simulink library "PowerFlowLib"  (Simulink 8.1)
settings: Solver=ode45  StartTime=0.0  StopTime=10.0  RelTol=1e-3
undefined symbols (not defined in the file or in its folder): Air, AirProp, C, F1, F2, Fanmap, Fld1, Fld2, Fluid, fueltankdata, HydProp, HydraulicLoad, IBFD_exc, L, LoadFluidProps, magnitude, MSSN, n_alghts, PumpProp, pwr_alghts, R_fd_exc, Rcore, Ts, VBFD_exc
libraries: PowerFlowLib x35, simulink x19, powerlib_extras x2, dspstat3 x2
(part 10 of 12)

== system PowerFlowLib/Energy & Power Systems/Electrical/Machines/Synchronous Machine P.U. dq0/Generator Power Loss ==
  Ed : Inport
  Eq : Inport  Port=2
  Id : Inport  Port=3
  Iq : Inport  Port=4
  Te : Inport  Port=5
  w/ws : Inport  Port=6
  Bus Creator : BusCreator  Inputs=6
  Gain1 : Gain  Gain=SB
  Gain2 : Gain  Gain=SB
  Gain3 : Gain  Gain=SB
  Product : Product  RndMeth=Zero
  Product1 : Product  RndMeth=Zero
  Product2 : Product  RndMeth=Zero
  Sum1 : Sum  Inputs=-+
  Sum2 : Sum
  PE : Outport
  PM : Outport  Port=2
  PLOSS : Outport  Port=3
  m : Outport  Port=4
  wires:
  Gain3/1 -> PM/1
  Gain1/1 -> PE/1
  Gain2/1 -> PLOSS/1
  Bus Creator/1 -> m/1
  [nu] -> Bus Creator/6  "nu"
  [Te] -> Bus Creator/5  "Te"
  [Iq] -> Bus Creator/4  "Iq"
  [Eq] -> Bus Creator/3  "Vq"
  [Id] -> Bus Creator/2  "Id"
  [Ed] -> Bus Creator/1  "Vd"
  Sum1/1 -> Gain2/1
  Product2/1 -> Gain3/1, Sum1/2
  Sum2/1 -> Gain1/1, Sum1/1
  Product1/1 -> Sum2/2
  Product/1 -> Sum2/1
  [nu] -> Product2/2
  [Te] -> Product2/1
  [Iq] -> Product1/2
  [Eq] -> Product1/1
  [Id] -> Product/2
  [Ed] -> Product/1
  w/ws/1 -> [nu]
  Te/1 -> [Te]
  Iq/1 -> [Iq]
  Id/1 -> [Id]
  Eq/1 -> [Eq]
  Ed/1 -> [Ed]

== system PowerFlowLib/Energy & Power Systems/Electrical/Machines/Synchronous Machine P.U. dq0/Generator Power Loss1 ==
  Ploss : Inport
  Tamb : Inport  Port=2
  Gain1 : Gain  Gain=1/mc_gen
  Heat Trasnfer : Subsystem
  Integrator : Integrator  InitialConditionSource=external
  Sum : Sum  Inputs=|+-
  Ts : Outport
  Pdiss : Outport  Port=2
  wires:
  Gain1/1 -> Integrator/1
  Heat Trasnfer/1(Pdiss) -> Pdiss/1, Sum/2
  Ploss/1 -> Sum/1
  Sum/1 -> Gain1/1
  Integrator/1 -> Heat Trasnfer/2(Ts), Ts/1
  Tamb/1 -> Heat Trasnfer/1(Tamb), Integrator/2

== system PowerFlowLib/Energy & Power Systems/Electrical/Machines/Synchronous Machine P.U. dq0/Stator Voltage ==
  Id : Inport
  Iq : Inport  Port=2
  Eq1 : Inport  Port=3
  Ed1 : Inport  Port=4
  Phi_1d : Inport  Port=5
  Phi_2q : Inport  Port=6
  w/ws : Inport  Port=7
  Gain : Gain  Gain=(Xq2 - Xls)/(Xq1 - Xls)
  Gain1 : Gain  Gain=(Xq1 - Xq2)/(Xq1 - Xls)
  Gain2 : Gain  Gain=(Xq2 - Xd2)
  Gain3 : Gain  Gain=(Xd2 - Xls)/(Xd1 - Xls)
  Gain4 : Gain  Gain=(Xd1 - Xd2)/(Xd1 - Xls)
  Gain5 : Gain  Gain=Rs
  Gain6 : Gain  Gain=Xd2+XTL
  Gain7 : Gain  Gain=Rs+RTL
  Gain8 : Gain  Gain=Xd2+XTL
  Product{,1..3} (4 alike) : Product  RndMeth=Zero
  Sum : Sum
  Sum1 : Sum  Inputs=+-+
  Sum2 : Sum  Inputs=--+
  Sum3 : Sum  Inputs=-++
  Ed : Outport
  Eq : Outport  Port=2
  wires:
  Gain7/1 -> Sum2/2
  Product3/1 -> Sum2/1
  Sum2/1 -> Eq/1  "Vq"
  Sum3/1 -> Ed/1  "Vd"
  Product2/1 -> Sum3/3
  Gain2/1 -> Sum1/3
  Product1/1 -> Sum3/2
  Gain8/1 -> Product3/1
  Gain5/1 -> Sum3/1
  Gain6/1 -> Product2/2
  Id/1 -> Gain8/1, Gain5/1
  Product/1 -> Sum2/3
  w/ws/1 -> Product2/1, Product3/2, Product/2, Product1/2
  Sum1/1 -> Product1/1
  Sum/1 -> Product/1
  Gain1/1 -> Sum1/2
  Gain/1 -> Sum1/1
  Gain3/1 -> Sum/1
  Gain4/1 -> Sum/2
  Phi_1d/1 -> Gain4/1
  Eq1/1 -> Gain3/1
  Iq/1 -> Gain2/1, Gain7/1, Gain6/1
  Phi_2q/1 -> Gain1/1
  Ed1/1 -> Gain/1

== system PowerFlowLib/Energy & Power Systems/Electrical/Systems/Gen Bus w/ APU switch/VOLTAGE FAULT DETECTION LOGIC ==
  note: This input determines the start of voltage monitoring
  In1 : Inport
  Constant1 : Constant  Value=LOWVLIMIT
  Constant2 : Constant  Value=UPVLIMIT
  Logical Operator : Logic  Operator=OR  AllPortsSameDT=off  OutDataTypeStr=boolean
  Logical Operator1 : Logic  Operator=NAND  AllPortsSameDT=off  OutDataTypeStr=boolean
  Relational Operator : RelationalOperator  Operator=<=  OutDataTypeStr=boolean  ZeroCross=off
  Relational Operator1 : RelationalOperator  OutDataTypeStr=boolean  ZeroCross=off
  Fault Signal  (Acitve Low) : Outport
  wires:
  Logical Operator1/1 -> Fault Signal  (Acitve Low)/1
  In1/1 -> Relational Operator1/1, Relational Operator/1
  [enable] -> Logical Operator1/2
  Logical Operator/1 -> Logical Operator1/1
  Relational Operator1/1 -> Logical Operator/2
  Relational Operator/1 -> Logical Operator/1
  Constant2/1 -> Relational Operator1/2
  Constant1/1 -> Relational Operator/2

== system PowerFlowLib/Energy & Power Systems/Electrical/Systems/Generation Unit Sync-Sync/Chopper (Averaged) ==
  vin : Inport
  q : Inport  Port=2
  Temperature : Inport  Port=3
  1/R : Gain  Gain=1/(R_fd_exc*VBFD_exc/IBFD_exc)/100/2*3/100  SaturateOnIntegerOverflow=on  OutDataTypeStr=Inherit: Same as input  ParamDataTypeStr=Inherit: Same as input
  Divide : Product  Inputs=*/
  Dot Product : DotProduct  InputSameDT=on  OutDataTypeStr=Inherit: Inherit via internal rule
  Dot Product1 : DotProduct  InputSameDT=on  OutDataTypeStr=Inherit: Inherit via internal rule
  Gain2 : Gain  Gain=1000*2/3
  Saturation : Saturate  UpperLimit=1  LowerLimit=0
  iout : Outport
  iin : Outport  Port=2
  wires:
  Dot Product1/1 -> iin/1
  Saturation/1 -> Dot Product1/2, Dot Product/2
  Dot Product/1 -> 1/R/1
  q/1 -> Saturation/1
  vin/1 -> Dot Product/1
  Gain2/1 -> Dot Product1/1, iout/1
  1/R/1 -> Divide/1
  Temperature/1 -> Divide/2
  Divide/1 -> Gain2/1

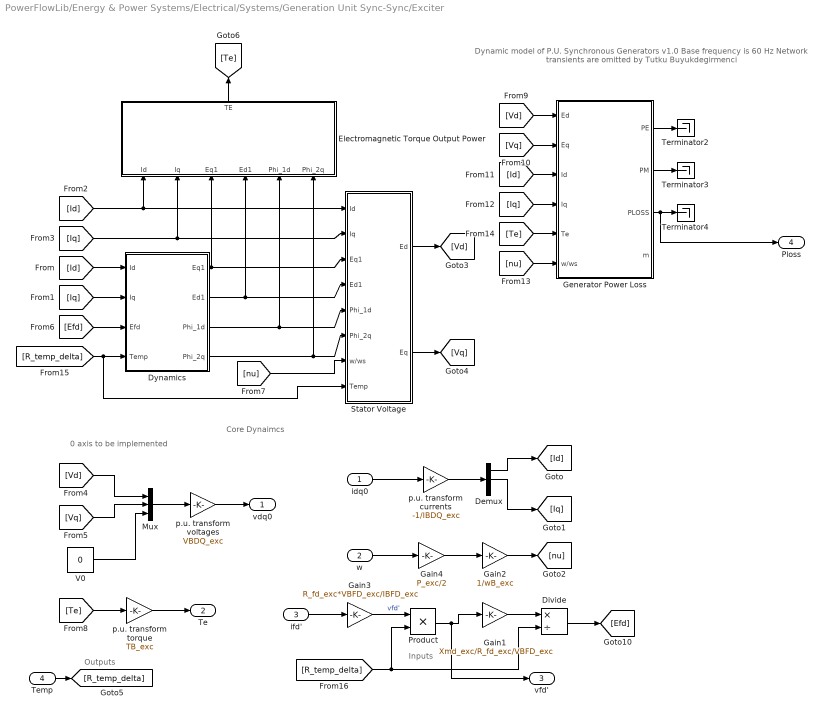
== system PowerFlowLib/Energy & Power Systems/Electrical/Systems/Generation Unit Sync-Sync/Exciter ==
  note: 0 axis to be implemented
  note: Inputs
  note: Outputs
  note: Core Dynaimcs
  note: Dynamic model of P.U. Synchronous Generators v1.0
      | Base frequency is 60 Hz
      | Network transients are omitted
      | by Tutku Buyukdegirmenci
  idq0 : Inport
  w : Inport  Port=2
  ifd' : Inport  Port=3
  Temp : Inport  Port=4
  Demux : Demux  Outputs=3
  Divide : Product  Inputs=*/
  Dynamics : Subsystem
  Electromagnetic Torque Output Power : Subsystem
  Gain1 : Gain  Gain=Xmd_exc/R_fd_exc/VBFD_exc
  Gain2 : Gain  Gain=1/wB_exc
  Gain3 : Gain  Gain=R_fd_exc*VBFD_exc/IBFD_exc
  Gain4 : Gain  Gain=P_exc/2
  Generator Power Loss : Subsystem
  Mux : Mux  Inputs=3
  Product : Product
  Stator Voltage : Subsystem
  Terminator2 : Terminator
  Terminator3 : Terminator
  Terminator4 : Terminator
  V0 : Constant  Value=0
  p.u. transform currents : Gain  Gain=-1/IBDQ_exc
  p.u. transform torque : Gain  Gain=TB_exc
  p.u. transform voltages : Gain  Gain=VBDQ_exc
  vdq0 : Outport
  Te : Outport  Port=2
  vfd' : Outport  Port=3
  Ploss : Outport  Port=4
  wires:
  Dynamics/1(Eq1) -> Stator Voltage/3(Eq1), Electromagnetic Torque Output Power/3(Eq1)
  Dynamics/2(Ed1) -> Stator Voltage/4(Ed1), Electromagnetic Torque Output Power/4(Ed1)
  Dynamics/3(Phi_1d) -> Stator Voltage/5(Phi_1d), Electromagnetic Torque Output Power/5(Phi_1d)
  Dynamics/4(Phi_2q) -> Stator Voltage/6(Phi_2q), Electromagnetic Torque Output Power/6(Phi_2q)
  Stator Voltage/2(Eq) -> [Vq]
  Stator Voltage/1(Ed) -> [Vd]
  w/1 -> Gain4/1
  Demux/1 -> [Id]
  Demux/2 -> [Iq]
  Gain2/1 -> [nu]
  [Id] -> Dynamics/1(Id)
  [Iq] -> Dynamics/2(Iq)
  [Id] -> Stator Voltage/1(Id), Electromagnetic Torque Output Power/1(Id)
  [Iq] -> Stator Voltage/2(Iq), Electromagnetic Torque Output Power/2(Iq)
  Mux/1 -> p.u. transform voltages/1
  [Vd] -> Mux/1
  [Vq] -> Mux/2
  V0/1 -> Mux/3
  [nu] -> Stator Voltage/7(w/ws)
  Electromagnetic Torque Output Power/1(TE) -> [Te]
  [Te] -> p.u. transform torque/1
  p.u. transform currents/1 -> Demux/1
  p.u. transform torque/1 -> Te/1
  [Vd] -> Generator Power Loss/1(Ed)
  [Vq] -> Generator Power Loss/2(Eq)
  [Id] -> Generator Power Loss/3(Id)
  [Iq] -> Generator Power Loss/4(Iq)
  [nu] -> Generator Power Loss/6(w/ws)
  [Te] -> Generator Power Loss/5(Te)
  Generator Power Loss/1(PE) -> Terminator2/1
  Generator Power Loss/2(PM) -> Terminator3/1
  Generator Power Loss/3(PLOSS) -> Ploss/1, Terminator4/1
  p.u. transform voltages/1 -> vdq0/1
  idq0/1 -> p.u. transform currents/1
  ifd'/1 -> Gain3/1
  [Efd] -> Dynamics/3(Efd)
  Gain4/1 -> Gain2/1
  Temp/1 -> [R_temp_delta]
  [R_temp_delta] -> Stator Voltage/8(Temp), Dynamics/4(Temp)
  Gain3/1 -> Product/1  "vfd'"
  Gain1/1 -> Divide/1
  Divide/1 -> [Efd]
  Product/1 -> vfd'/1, Gain1/1
  [R_temp_delta] -> Product/2, Divide/2

== system PowerFlowLib/Energy & Power Systems/Electrical/Systems/Generation Unit Sync-Sync/Generator ==
  note: Dynamic model of P.U. Synchronous Generators v1.0
      | Base frequency is 60 Hz
      | Network transients are omitted
      | by Tutku Buyukdegirmenci
  note: Core Dynaimcs
  note: Outputs
  note: Inputs
  note: 0 axis to be implemented
  idq0 : Inport
  w : Inport  Port=2
  ifd' : Inport  Port=3
  Temp : Inport  Port=4
  Demux : Demux  Outputs=3
  Divide : Product  Inputs=*/
  Dynamics : Subsystem
  Electromagnetic Torque Output Power : Subsystem
  Gain1 : Gain  Gain=Xmd/R_fd/VBFD
  Gain2 : Gain  Gain=1/wB
  Gain3 : Gain  Gain=R_fd*VBFD/IBFD
  Gain4 : Gain  Gain=P/2
  Generator Power Loss : Subsystem
  Mux : Mux  Inputs=3
  Product : Product
  Stator Voltage : Subsystem
  Terminator2 : Terminator
  Terminator3 : Terminator
  Terminator4 : Terminator
  V0 : Constant  Value=0
  p.u. transform currents : Gain  Gain=-1/IBDQ
  p.u. transform torque : Gain  Gain=TB
  p.u. transform voltages : Gain  Gain=VBDQ
  vdq0 : Outport
  Te : Outport  Port=2
  vfd' : Outport  Port=3
  Ploss : Outport  Port=4
  wires:
  Gain4/1 -> Gain2/1
  [Efd] -> Dynamics/3(Efd)
  ifd'/1 -> Gain3/1
  idq0/1 -> p.u. transform currents/1
  p.u. transform voltages/1 -> vdq0/1
  Generator Power Loss/3(PLOSS) -> Ploss/1, Terminator4/1
  Generator Power Loss/2(PM) -> Terminator3/1
  Generator Power Loss/1(PE) -> Terminator2/1
  [Te] -> Generator Power Loss/5(Te)
  [nu] -> Generator Power Loss/6(w/ws)
  [Iq] -> Generator Power Loss/4(Iq)
  [Id] -> Generator Power Loss/3(Id)
  [Vq] -> Generator Power Loss/2(Eq)
  [Vd] -> Generator Power Loss/1(Ed)
  p.u. transform torque/1 -> Te/1
  p.u. transform currents/1 -> Demux/1
  [Te] -> p.u. transform torque/1
  Electromagnetic Torque Output Power/1(TE) -> [Te]
  [nu] -> Stator Voltage/7(w/ws)
  V0/1 -> Mux/3
  [Vq] -> Mux/2
  [Vd] -> Mux/1
  Mux/1 -> p.u. transform voltages/1
  [Iq] -> Electromagnetic Torque Output Power/2(Iq), Stator Voltage/2(Iq)
  [Id] -> Electromagnetic Torque Output Power/1(Id), Stator Voltage/1(Id)
  [Iq] -> Dynamics/2(Iq)
  [Id] -> Dynamics/1(Id)
  Gain2/1 -> [nu]
  Demux/2 -> [Iq]
  Demux/1 -> [Id]
  w/1 -> Gain4/1
  Stator Voltage/1(Ed) -> [Vd]
  Stator Voltage/2(Eq) -> [Vq]
  Dynamics/4(Phi_2q) -> Electromagnetic Torque Output Power/6(Phi_2q), Stator Voltage/6(Phi_2q)
  Dynamics/3(Phi_1d) -> Electromagnetic Torque Output Power/5(Phi_1d), Stator Voltage/5(Phi_1d)
  Dynamics/2(Ed1) -> Electromagnetic Torque Output Power/4(Ed1), Stator Voltage/4(Ed1)
  Dynamics/1(Eq1) -> Electromagnetic Torque Output Power/3(Eq1), Stator Voltage/3(Eq1)
  Temp/1 -> [R_temp_delta]
  Gain1/1 -> Divide/1
  Divide/1 -> [Efd]
  Gain3/1 -> Product/1  "vfd'"
  Product/1 -> Gain1/1, vfd'/1
  [R_temp_delta] -> Divide/2, Product/2
  [R_temp_delta] -> Stator Voltage/8(Temp), Dynamics/4(Temp)

== system PowerFlowLib/Energy & Power Systems/Electrical/Systems/Generator Bus/Compare To Constant ==
  u : Inport
  Compare : RelationalOperator  Operator===  OutDataTypeStr=fixdt(0, 8)  InputSameDT=on
  Constant : Constant  DisableCoverage=on  Value=const  OutDataTypeStr=Inherit: Inherit via back propagation
  y : Outport
  wires:
  u/1 -> Compare/1
  Constant/1 -> Compare/2
  Compare/1 -> y/1

== system PowerFlowLib/Energy & Power Systems/Electrical/Systems/Generator Bus/Compare To Constant1 ==
  u : Inport
  Compare : RelationalOperator  Operator===  OutDataTypeStr=fixdt(0, 8)  InputSameDT=on
  Constant : Constant  DisableCoverage=on  Value=const  OutDataTypeStr=Inherit: Inherit via back propagation
  y : Outport
  wires:
  u/1 -> Compare/1
  Constant/1 -> Compare/2
  Compare/1 -> y/1

== system PowerFlowLib/Energy & Power Systems/Electrical/Systems/Generator Bus/Compare To Constant2 ==
  u : Inport
  Compare : RelationalOperator  Operator===  OutDataTypeStr=fixdt(0, 8)  InputSameDT=on
  Constant : Constant  DisableCoverage=on  Value=const  OutDataTypeStr=Inherit: Inherit via back propagation
  y : Outport
  wires:
  u/1 -> Compare/1
  Constant/1 -> Compare/2
  Compare/1 -> y/1

== system PowerFlowLib/Energy & Power Systems/Electrical/Systems/Generator Bus/Compare To Constant3 ==
  u : Inport
  Compare : RelationalOperator  Operator===  OutDataTypeStr=fixdt(0, 8)  InputSameDT=on
  Constant : Constant  DisableCoverage=on  Value=const  OutDataTypeStr=Inherit: Inherit via back propagation
  y : Outport
  wires:
  u/1 -> Compare/1
  Constant/1 -> Compare/2
  Compare/1 -> y/1

== system PowerFlowLib/Energy & Power Systems/Electrical/Systems/three-phase  full-bridge  inverter/Three-Phase Full Bridge Inverter CONSTANT FREQUENCY1 ==
  Vdc : Inport
  Inverter current : Inport  Port=2
  Add : Sum
  Constant : Constant  Value=Tr
  Constant1 : Constant  Value=Tf
  Constant2 : Constant  Value=Fsw
  Constant3 : Constant  Value=VCEsat
  Display : Display
  No. of IGBT switches : Gain  Gain=Nsw
  "No. of series vol drops " : Gain  Gain=3
  Product : Product  RndMeth=Zero
  Switch Loss : Subsystem
  Total Loss : Outport
  Switching Loss : Outport  Port=2
  Conduction Loss : Outport  Port=3
  wires:
  Product/1 -> Conduction Loss/1, Add/2
  No. of IGBT switches/1 -> Switching Loss/1, Add/1
  Add/1 -> Total Loss/1
  "No. of series vol drops "/1 -> Product/2
  Constant3/1 -> "No. of series vol drops "/1
  Vdc/1 -> Switch Loss/1(Vdc)
  Constant2/1 -> Switch Loss/5(Fsw mean)
  Switch Loss/1(Switch Loss) -> No. of IGBT switches/1
  Inverter current/1 -> Product/1, Switch Loss/4(Inverter phase current)
  Constant1/1 -> Switch Loss/3(Tfall)
  Constant/1 -> Switch Loss/2(Trise)

== system PowerFlowLib/Energy & Power Systems/Thermal/ECS/ACM/Compressor ==
  Flow In : Inport
  omega_rad/s : Inport  Port=2
  Bias : Bias
  Bias1 : Bias
  Bus Creator : BusCreator  Inputs=2
  Bus Selector : BusSelector  OutputSignals=mdot_kgps,temp_K
  Constant : Constant  Value=Comp_r2
  Fcn : Fcn  Expr=u(1)^2*u(2)^2/Air.cp
  Gain : Gain  Gain=Air.cp
  Mux : Mux  Inputs=2
  Product : Product
  Sum : Sum  Inputs=|++
  Sum1 : Sum  Inputs=|+-
  "Flow Out " : Outport
  Power [W] : Outport  Port=2
  wires:
  omega_rad/s/1 -> Mux/1
  Mux/1 -> Fcn/1
  Fcn/1 -> Sum/2
  Constant/1 -> Mux/2
  Sum1/1 -> Gain/1
  Product/1 -> Power [W]/1
  Gain/1 -> Product/2
  Flow In/1 -> Bus Selector/1
  Bus Selector/1 -> Product/1, Bus Creator/2  "<mdot_kgps>"
  Bus Selector/2 -> Bias/1  "<temp_K>"
  Sum/1 -> Bias1/1, Sum1/2  "T_K"
  Bus Creator/1 -> "Flow Out "/1
  Bias/1 -> Sum/1, Sum1/1
  Bias1/1 -> Bus Creator/1  "temp_K"

== system PowerFlowLib/Energy & Power Systems/Thermal/ECS/ACM/Expanding Turbine ==
  Flow In : Inport
  omega_rad/s : Inport  Port=2
  Bias : Bias
  Bias1 : Bias
  Bus Creator : BusCreator  Inputs=3
  Bus Selector : BusSelector  OutputSignals=mdot_kgps,temp_K
  Constant : Constant  Value=Turb_r1
  Constant1 : Constant  Value=101
  Fcn : Fcn  Expr=u(1)^2*u(2)^2/Air.cp
  Gain : Gain  Gain=Air.cp*0.85
  Mux : Mux  Inputs=2
  Product : Product
  Sum : Sum  Inputs=|+-
  Sum1 : Sum  Inputs=|+-
  Power [W] : Outport
  Flow Out : Outport  Port=2
  wires:
  Gain/1 -> Product/2
  Product/1 -> Power [W]/1
  Sum1/1 -> Gain/1
  Constant/1 -> Mux/2
  Fcn/1 -> Sum/2
  Mux/1 -> Fcn/1
  omega_rad/s/1 -> Mux/1
  Sum/1 -> Bias1/1, Sum1/2  "T_K"
  Bus Creator/1 -> Flow Out/1  "Flow Out"
  Flow In/1 -> Bus Selector/1
  Bus Selector/1 -> Bus Creator/2, Product/1  "<mdot_kgps>"
  Bus Selector/2 -> Bias/1  "<temp_K>"
  Bias/1 -> Sum/1, Sum1/1
  Bias1/1 -> Bus Creator/1  "temp_K"
  Constant1/1 -> Bus Creator/3  "pres_kPa"

== system PowerFlowLib/Energy & Power Systems/Thermal/ECS/ACM/Power Turbine ==
  Flow In : Inport
  temp_3rd : Inport  Port=2
  Bias : Bias
  Bus Creator : BusCreator  Inputs=2
  Bus Selector : BusSelector  OutputSignals=mdot_kgps,temp_K
  Gain : Gain  Gain=Air.cp
  Product : Product
  Sum1 : Sum  Inputs=|+-
  Power [W] : Outport
  Flow Out : Outport  Port=2
  wires:
  Bus Selector/2 -> Sum1/1  "<temp_K>"
  Bus Selector/1 -> Product/1, Bus Creator/2  "<mdot_kgps>"
  Flow In/1 -> Bus Selector/1
  Bus Creator/1 -> Flow Out/1
  temp_3rd/1 -> Bias/1  "T_K"
  Sum1/1 -> Gain/1
  Product/1 -> Power [W]/1
  Gain/1 -> Product/2
  Bias/1 -> Sum1/2, Bus Creator/1

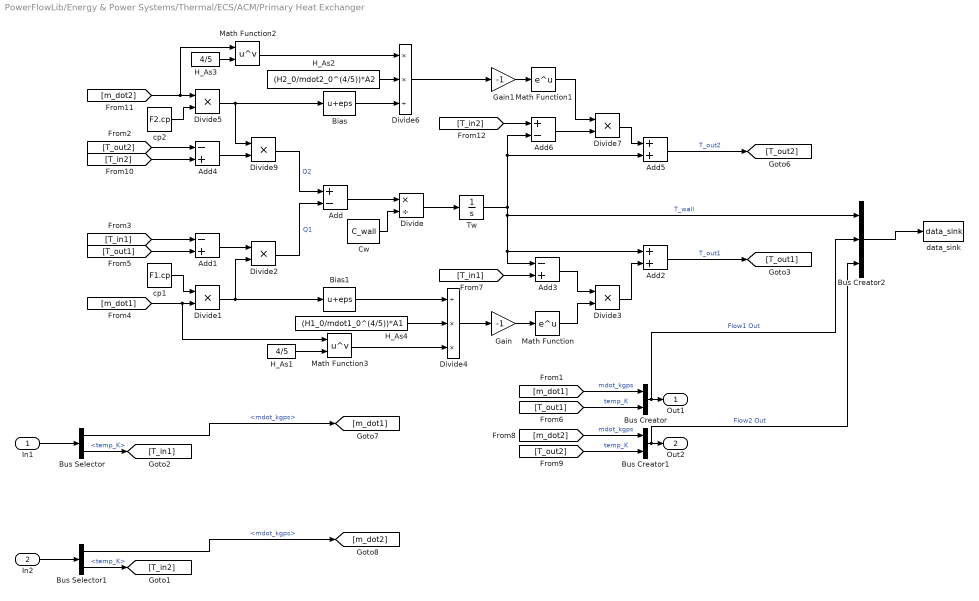
== system PowerFlowLib/Energy & Power Systems/Thermal/ECS/ACM/Primary Heat Exchanger ==
  In1 : Inport
  In2 : Inport  Port=2
  Add : Sum  Inputs=+-
  Add1 : Sum  Inputs=-+
  Add2 : Sum
  Add3 : Sum  Inputs=-+
  Add4 : Sum  Inputs=-+
  Add5 : Sum
  Add6 : Sum  Inputs=+-
  Bias : Bias  Bias=eps
  Bias1 : Bias  Bias=eps
  Bus Creator : BusCreator  Inputs=2
  Bus Creator1 : BusCreator  Inputs=2
  Bus Creator2 : BusCreator  Inputs=3
  Bus Selector : BusSelector  OutputSignals=mdot_kgps,temp_K
  Bus Selector1 : BusSelector  OutputSignals=mdot_kgps,temp_K
  Cw : Constant  Value=C_wall
  Divide : Product  Inputs=*/
  Divide{1..3,5,7,9} (6 alike) : Product  Inputs=**
  Divide4 : Product  Inputs=/**
  Divide6 : Product  Inputs=**/
  Gain : Gain  Gain=-1
  Gain1 : Gain  Gain=-1
  H_As1 : Constant  Value=4/5
  H_As2 : Constant  Value=(H2_0/mdot2_0^(4/5))*A2
  H_As3 : Constant  Value=4/5
  H_As4 : Constant  Value=(H1_0/mdot1_0^(4/5))*A1
  Math Function : Math  SaturateOnIntegerOverflow=on
  Math Function1 : Math  SaturateOnIntegerOverflow=on
  Math Function2 : Math  Operator=pow  SaturateOnIntegerOverflow=on
  Math Function3 : Math  Operator=pow  SaturateOnIntegerOverflow=on
  Tw : Integrator  InitialCondition=Tw_init+273.15
  cp1 : Constant  Value=F1.cp
  cp2 : Constant  Value=F2.cp
  data_sink : PowerFlowLib/Support Functions//Tools/data_sink
  Out1 : Outport
  Out2 : Outport  Port=2
  wires:
  Bus Creator2/1 -> data_sink/1
  H_As1/1 -> Math Function3/2
  Math Function3/1 -> Divide4/3
  H_As3/1 -> Math Function2/2
  Math Function2/1 -> Divide6/1
  Cw/1 -> Divide/2
  Add/1 -> Divide/1
  In1/1 -> Bus Selector/1
  cp1/1 -> Divide1/1
  Add2/1 -> [T_out1]  "T_out1"
  Divide2/1 -> Add/2  "Q1"
  Tw/1 -> Add6/2, Add5/2, Add2/1, Add3/1, Bus Creator2/1  "T_wall"
  Divide3/1 -> Add2/2
  Add3/1 -> Divide3/1
  Bus Creator/1 -> Out1/1, Bus Creator2/2  "Flow1 Out"
  [m_dot1] -> Bus Creator/1  "mdot_kgps"
  Divide9/1 -> Add/1  "Q2"
  Bus Selector/2 -> [T_in1]  "<temp_K>"
  [T_in1] -> Add1/1
  [m_dot1] -> Divide1/2, Math Function3/1
  [T_out1] -> Add1/2
  [T_out1] -> Bus Creator/2  "temp_K"
  [T_in1] -> Add3/2
  Math Function/1 -> Divide3/2
  Add1/1 -> Divide2/1
  Divide1/1 -> Divide2/2, Bias1/1
  Divide4/1 -> Gain/1
  H_As4/1 -> Divide4/2
  Gain/1 -> Math Function/1
  In2/1 -> Bus Selector1/1
  Bus Selector1/2 -> [T_in2]  "<temp_K>"
  Bus Creator1/1 -> Out2/1, Bus Creator2/3  "Flow2 Out"
  [m_dot2] -> Bus Creator1/1  "mdot_kgps"
  [T_out2] -> Bus Creator1/2  "temp_K"
  Add4/1 -> Divide9/2
  [T_in2] -> Add4/2
  [T_out2] -> Add4/1
  Divide5/1 -> Bias/1, Divide9/1
  cp2/1 -> Divide5/2
  [m_dot2] -> Divide5/1, Math Function2/1
  H_As2/1 -> Divide6/2
  Divide6/1 -> Gain1/1
  Gain1/1 -> Math Function1/1
  Math Function1/1 -> Divide7/1
  Add5/1 -> [T_out2]  "T_out2"
  Divide7/1 -> Add5/1
  Add6/1 -> Divide7/2
  [T_in2] -> Add6/1
  Bus Selector/1 -> [m_dot1]  "<mdot_kgps>"
  Bus Selector1/1 -> [m_dot2]  "<mdot_kgps>"
  Bias/1 -> Divide6/3
  Bias1/1 -> Divide4/1
  Divide/1 -> Tw/1

== system PowerFlowLib/Energy & Power Systems/Thermal/ECS/ACM/Shaft ==
  Power In/Out [vector] : Inport
  Bus Creator2 : BusCreator  Inputs=1
  Comp Inertia : Constant  Value=J_comp
  Divide : Product  Inputs=*//
  Integrator : Integrator  InitialCondition=N_init * 2 * pi / 60 + eps  LimitOutput=on  LowerSaturationLimit=0
  Mux : Mux
  Pwr Turb Inertia : Constant  Value=J_pturb
  Shaft Inertia : Constant  Value=J_shaft
  Sum of Elements : Sum  Inputs=+
  Sum of Elements1 : Sum  Inputs=+
  Turb Inertia : Constant  Value=J_turb
  data_sink : PowerFlowLib/Support Functions//Tools/data_sink
  rad 2 rev : Gain  Gain=60/2/pi
  Angular Velocity [rad/s] : Outport
  wires:
  Integrator/1 -> Divide/3, rad 2 rev/1, Angular Velocity [rad/s]/1  "omega (rad/s)"
  Power In/Out [vector]/1 -> Sum of Elements/1
  Sum of Elements/1 -> Divide/1
  Divide/1 -> Integrator/1
  Sum of Elements1/1 -> Divide/2
  Shaft Inertia/1 -> Mux/1
  Comp Inertia/1 -> Mux/2
  Turb Inertia/1 -> Mux/3
  Pwr Turb Inertia/1 -> Mux/4
  Mux/1 -> Sum of Elements1/1
  rad 2 rev/1 -> Bus Creator2/1  "RPM"
  Bus Creator2/1 -> data_sink/1

== system PowerFlowLib/Energy & Power Systems/Thermal/ECS/ACM/Signal Routing ==
  Flow In : Inport
  Bus Creator : BusCreator  Inputs=2
  Bus Selector : BusSelector  OutputSignals=temp_K,mdot_kgps
  Flow Out : Outport
  wires:
  Flow In/1 -> Bus Selector/1
  Bus Selector/1 -> Bus Creator/1  "<temp_K>"
  Bus Selector/2 -> Bus Creator/2  "<mdot_kgps>"
  Bus Creator/1 -> Flow Out/1

== system PowerFlowLib/Energy & Power Systems/Thermal/ECS/Air-Air HX/Air_properties_in_flows_hot_and_cold ==
  In_flow_bus_hot : Inport
  In_flow_bus_cold : Inport  Port=2
  Bus Creator : BusCreator  Inputs=5
  Bus Creator3 : BusCreator  Inputs=5
  air_properties_in_cold : Subsystem
  air_properties_in_hot : Subsystem
  air_properties_in_hot1 : Outport
  air_properties_in_cold1 : Outport  Port=2
  wires:
  air_properties_in_hot/4(K_air_Wm-1K-2) -> Bus Creator/4  "K_air"
  air_properties_in_cold/5(Pr) -> Bus Creator3/5  "Pr"
  air_properties_in_hot/5(Pr) -> Bus Creator/5  "Pr"
  In_flow_bus_cold/1 -> air_properties_in_cold/1(In_flow_bus_cold)
  In_flow_bus_hot/1 -> air_properties_in_hot/1(In_flow_bus_hot)
  Bus Creator/1 -> air_properties_in_hot1/1
  Bus Creator3/1 -> air_properties_in_cold1/1
  air_properties_in_hot/3(mu_air_Pa.s) -> Bus Creator/3  "mu_air"
  air_properties_in_hot/2(cp_air_Jkg-1K-1) -> Bus Creator/2  "cp_air"
  air_properties_in_hot/1(rho_air_kgm-3) -> Bus Creator/1  "rho_air"
  air_properties_in_cold/4(K_air_Wm-1K-2) -> Bus Creator3/4  "K_air"
  air_properties_in_cold/3(mu_air_Pa.s) -> Bus Creator3/3  "mu_air"
  air_properties_in_cold/2(cp_air_Jkg-1K-1) -> Bus Creator3/2  "cp_air"
  air_properties_in_cold/1(rho_air_kgm-3) -> Bus Creator3/1  "rho_air"

== system PowerFlowLib/Energy & Power Systems/Thermal/ECS/Air-Air HX/C_T_c_av ==
  In_flow_bus : Inport
  air_properties : Inport  Port=2
  Tot_thermal_resist : Inport  Port=3
  Add : Sum
  Bus Selector : BusSelector  OutputSignals=mdot_kgps
  Bus Selector1 : BusSelector  OutputSignals=cp_air
  Constant : Constant
  Divide : Product  Inputs=***
  Divide1 : Product  Inputs=*/
  Gain : Gain  Gain=2
  C_T_c_av : Outport
  wires:
  Divide1/1 -> C_T_c_av/1
  Add/1 -> Divide1/2
  Constant/1 -> Add/2
  Gain/1 -> Divide1/1, Add/1
  Divide/1 -> Gain/1
  Bus Selector1/1 -> Divide/3  "<cp_air>"
  Bus Selector/1 -> Divide/2  "<mdot_kgps>"
  Tot_thermal_resist/1 -> Divide/1  "R_tot_c"
  In_flow_bus/1 -> Bus Selector/1
  air_properties/1 -> Bus Selector1/1

== system PowerFlowLib/Energy & Power Systems/Thermal/ECS/Air-Air HX/C_T_c_i ==
  In_flow_bus : Inport
  air_properties : Inport  Port=2
  Tot_thermal_resist : Inport  Port=3
  HX_parameters : Inport  Port=4
  Add : Sum
  Bus Selector : BusSelector  OutputSignals=mdot_kgps
  Bus Selector1 : BusSelector  OutputSignals=cp_air
  Bus Selector2 : BusSelector  OutputSignals=m_cm,cp_hx
  Constant : Constant
  Divide : Product  Inputs=***
  Divide2 : Product  Inputs=**///
  Gain : Gain  Gain=2
  Gain1 : Gain  Gain=2
  C_T_c_i : Outport
  wires:
  In_flow_bus/1 -> Bus Selector/1
  air_properties/1 -> Bus Selector1/1
  Tot_thermal_resist/1 -> Divide/1  "R_tot"
  Bus Selector/1 -> Divide/2, Divide2/1  "<mdot_kgps>"
  Bus Selector1/1 -> Divide/3, Divide2/2  "<cp_air>"
  Divide/1 -> Gain/1
  Gain/1 -> Add/1
  Constant/1 -> Add/2
  HX_parameters/1 -> Bus Selector2/1
  Bus Selector2/1 -> Divide2/3  "<m_cm>"
  Bus Selector2/2 -> Divide2/4  "<cp_hx>"
  Add/1 -> Divide2/5
  Gain1/1 -> C_T_c_i/1
  Divide2/1 -> Gain1/1

== system PowerFlowLib/Energy & Power Systems/Thermal/ECS/Air-Air HX/C_T_h_av ==
  In_flow_bus : Inport
  air_properties : Inport  Port=2
  Tot_thermal_resist : Inport  Port=3
  Add : Sum
  Bus Selector : BusSelector  OutputSignals=mdot_kgps
  Bus Selector1 : BusSelector  OutputSignals=cp_air
  Constant : Constant
  Divide : Product  Inputs=***
  Divide1 : Product  Inputs=*/
  Gain : Gain  Gain=2
  C_T_h_av : Outport
  wires:
  Divide1/1 -> C_T_h_av/1
  Add/1 -> Divide1/2
  Constant/1 -> Add/2
  Gain/1 -> Divide1/1, Add/1
  Divide/1 -> Gain/1
  Bus Selector1/1 -> Divide/3  "<cp_air>"
  Bus Selector/1 -> Divide/2  "<mdot_kgps>"
  Tot_thermal_resist/1 -> Divide/1  "R_tot_h"
  In_flow_bus/1 -> Bus Selector/1
  air_properties/1 -> Bus Selector1/1

== system PowerFlowLib/Energy & Power Systems/Thermal/ECS/Air-Air HX/C_T_h_i ==
  In_flow_bus : Inport
  air_properties : Inport  Port=2
  Tot_thermal_resist : Inport  Port=3
  HX_parameters : Inport  Port=4
  Add : Sum
  Bus Selector : BusSelector  OutputSignals=mdot_kgps
  Bus Selector1 : BusSelector  OutputSignals=cp_air
  Bus Selector2 : BusSelector  OutputSignals=m_cm,cp_hx
  Constant : Constant
  Divide : Product  Inputs=***
  Divide2 : Product  Inputs=**///
  Gain : Gain  Gain=2
  Gain1 : Gain  Gain=2
  C_T_h_i : Outport
  wires:
  Gain1/1 -> C_T_h_i/1
  Add/1 -> Divide2/5
  Bus Selector2/2 -> Divide2/4  "<cp_hx>"
  Bus Selector2/1 -> Divide2/3  "<m_cm>"
  HX_parameters/1 -> Bus Selector2/1
  Constant/1 -> Add/2
  Gain/1 -> Add/1
  Divide/1 -> Gain/1
  Bus Selector1/1 -> Divide/3, Divide2/2  "<cp_air>"
  Bus Selector/1 -> Divide/2, Divide2/1  "<mdot_kgps>"
  Tot_thermal_resist/1 -> Divide/1  "R_tot_h"
  air_properties/1 -> Bus Selector1/1
  In_flow_bus/1 -> Bus Selector/1
  Divide2/1 -> Gain1/1

== system PowerFlowLib/Energy & Power Systems/Thermal/ECS/Air-Air HX/Calculating_T_c_av ==
  T_cm : Inport
  In_flow_bus : Inport  Port=2
  C_t_c_av : Inport  Port=3
  Add1 : Sum  Inputs=-+
  Add3 : Sum
  Bus Selector : BusSelector  OutputSignals=temp_C
  Divide1 : Product  Inputs=**
  T_c_av_degreC : Outport
  wires:
  T_cm/1 -> Add3/1, Add1/1  "T_cm"
  In_flow_bus/1 -> Bus Selector/1
  Bus Selector/1 -> Add1/2  "<temp_C>"
  C_t_c_av/1 -> Divide1/2
  Add1/1 -> Divide1/1  "T_c_i - T_cm"
  Divide1/1 -> Add3/2
  Add3/1 -> T_c_av_degreC/1

== system PowerFlowLib/Energy & Power Systems/Thermal/ECS/Air-Air HX/Calculating_T_h_av ==
  T_cm : Inport
  In_flow_bus : Inport  Port=2
  C_t_h_av : Inport  Port=3
  Add1 : Sum  Inputs=-+
  Add3 : Sum
  Bus Selector : BusSelector  OutputSignals=temp_C
  Divide1 : Product  Inputs=**
  T_h_av_degreC : Outport
  wires:
  Add1/1 -> Divide1/1  "T_h_i - T_cm"
  C_t_h_av/1 -> Divide1/2
  Bus Selector/1 -> Add1/2  "<temp_C>"
  In_flow_bus/1 -> Bus Selector/1
  T_cm/1 -> Add1/1, Add3/1  "T_cm"
  Add3/1 -> T_h_av_degreC/1
  Divide1/1 -> Add3/2

== system PowerFlowLib/Energy & Power Systems/Thermal/ECS/Air-Air HX/Calculating_core_mass_temp ==
  note: dTcm/dt
  note: Tcm
  C_T_h_i : Inport
  C_T_c_i : Inport  Port=2
  C_t_cm : Inport  Port=3
  In_flow_bus_hot : Inport  Port=4
  In_flow_bus_cold : Inport  Port=5
  Add : Sum  Inputs=++-
  Bus Selector : BusSelector  OutputSignals=temp_C
  Bus Selector1 : BusSelector  OutputSignals=temp_C
  Divide : Product  Inputs=**
  Divide1 : Product  Inputs=**
  Divide2 : Product  Inputs=**
  Integrator : Integrator  InitialCondition=T_cm_0
  Core_mass_temp_C : Outport
  wires:
  Divide1/1 -> Add/3
  C_t_cm/1 -> Divide1/2
  Integrator/1 -> Core_mass_temp_C/1, Divide1/1
  Add/1 -> Integrator/1
  Divide2/1 -> Add/2
  Divide/1 -> Add/1
  Bus Selector1/1 -> Divide2/2  "<temp_C>"
  C_T_c_i/1 -> Divide2/1
  Bus Selector/1 -> Divide/2  "<temp_C>"
  C_T_h_i/1 -> Divide/1
  In_flow_bus_cold/1 -> Bus Selector1/1
  In_flow_bus_hot/1 -> Bus Selector/1

== system PowerFlowLib/Energy & Power Systems/Thermal/ECS/Air-Air HX/Colburn_J_factor_cold ==
  Fin_prameter_ratios : Inport
  Re : Inport  Port=2
  Add : Sum
  Bus Selector : BusSelector  OutputSignals=alpha_fin,delta_fin,gamma_fin
  Constant : Constant  Value=-0.5403
  Constant1 : Constant  Value=-0.1541
  Constant2 : Constant  Value=0.1499
  Constant3 : Constant  Value=-0.0678
  Constant4 : Constant  Value=1.34
  Constant5 : Constant  Value=0.504
  Constant6 : Constant  Value=0.456
  Constant7 : Constant  Value=-1.055
  Constant8 : Constant
  Constant9 : Constant  Value=0.1
  Divide : Product  Inputs=****
  Divide1 : Product  Inputs=****
  Divide2 : Product  Inputs=**
  Gain : Gain  Gain=0.6522
  Gain1 : Gain  Gain=5.269*10^(-5)
  Re1 : Math  Operator=pow  SaturateOnIntegerOverflow=on
  Re2 : Math  Operator=pow  SaturateOnIntegerOverflow=on
  alpha_fin : Math  Operator=pow  SaturateOnIntegerOverflow=on
  alpha_fin1 : Math  Operator=pow  SaturateOnIntegerOverflow=on
  delta_fin : Math  Operator=pow  SaturateOnIntegerOverflow=on
  delta_fin1 : Math  Operator=pow  SaturateOnIntegerOverflow=on
  gamma_fin : Math  Operator=pow  SaturateOnIntegerOverflow=on
  gamma_fin1 : Math  Operator=pow  SaturateOnIntegerOverflow=on
  gamma_fin2 : Math  Operator=pow  SaturateOnIntegerOverflow=on
  Colburn_J_factor : Outport
  wires:
  Divide2/1 -> Colburn_J_factor/1
  Gain/1 -> Divide2/1
  gamma_fin2/1 -> Divide2/2
  Constant9/1 -> gamma_fin2/2
  Add/1 -> gamma_fin2/1
  Gain1/1 -> Add/1
  Constant8/1 -> Add/2
  Divide1/1 -> Gain1/1
  gamma_fin1/1 -> Divide1/4
  delta_fin1/1 -> Divide1/3
  alpha_fin1/1 -> Divide1/2
  Re2/1 -> Divide1/1
  Divide/1 -> Gain/1
  gamma_fin/1 -> Divide/4
  delta_fin/1 -> Divide/3
  alpha_fin/1 -> Divide/2
  Re1/1 -> Divide/1
  Bus Selector/3 -> gamma_fin1/1, gamma_fin/1  "<gamma_fin>"
  Bus Selector/2 -> delta_fin1/1, delta_fin/1  "<delta_fin>"
  Bus Selector/1 -> alpha_fin1/1, alpha_fin/1  "<alpha_fin>"
  Re/1 -> Re2/1, Re1/1
  Constant7/1 -> gamma_fin1/2
  Constant6/1 -> delta_fin1/2
  Constant5/1 -> alpha_fin1/2
  Constant4/1 -> Re2/2
  Constant3/1 -> gamma_fin/2
  Constant2/1 -> delta_fin/2
  Constant1/1 -> alpha_fin/2
  Constant/1 -> Re1/2
  Fin_prameter_ratios/1 -> Bus Selector/1

== system PowerFlowLib/Energy & Power Systems/Thermal/ECS/Air-Air HX/Colburn_J_factor_hot ==
  Fin_prameter_ratios : Inport
  Re : Inport  Port=2
  Add : Sum
  Bus Selector : BusSelector  OutputSignals=alpha_fin,delta_fin,gamma_fin
  Constant : Constant  Value=-0.5403
  Constant1 : Constant  Value=-0.1541
  Constant2 : Constant  Value=0.1499
  Constant3 : Constant  Value=-0.0678
  Constant4 : Constant  Value=1.34
  Constant5 : Constant  Value=0.504
  Constant6 : Constant  Value=0.456
  Constant7 : Constant  Value=-1.055
  Constant8 : Constant
  Constant9 : Constant  Value=0.1
  Divide : Product  Inputs=****
  Divide1 : Product  Inputs=****
  Divide2 : Product  Inputs=**
  Gain : Gain  Gain=0.6522
  Gain1 : Gain  Gain=5.269*10^(-5)
  Re1 : Math  Operator=pow  SaturateOnIntegerOverflow=on
  Re2 : Math  Operator=pow  SaturateOnIntegerOverflow=on
  alpha_fin : Math  Operator=pow  SaturateOnIntegerOverflow=on
  alpha_fin1 : Math  Operator=pow  SaturateOnIntegerOverflow=on
  delta_fin : Math  Operator=pow  SaturateOnIntegerOverflow=on
  delta_fin1 : Math  Operator=pow  SaturateOnIntegerOverflow=on
  gamma_fin : Math  Operator=pow  SaturateOnIntegerOverflow=on
  gamma_fin1 : Math  Operator=pow  SaturateOnIntegerOverflow=on
  gamma_fin2 : Math  Operator=pow  SaturateOnIntegerOverflow=on
  Colburn_J_factor : Outport
  wires:
  Fin_prameter_ratios/1 -> Bus Selector/1
  Constant/1 -> Re1/2
  Constant1/1 -> alpha_fin/2
  Constant2/1 -> delta_fin/2
  Constant3/1 -> gamma_fin/2
  Constant4/1 -> Re2/2
  Constant5/1 -> alpha_fin1/2
  Constant6/1 -> delta_fin1/2
  Constant7/1 -> gamma_fin1/2
  Re/1 -> Re1/1, Re2/1
  Bus Selector/1 -> alpha_fin/1, alpha_fin1/1  "<alpha_fin>"
  Bus Selector/2 -> delta_fin/1, delta_fin1/1  "<delta_fin>"
  Bus Selector/3 -> gamma_fin/1, gamma_fin1/1  "<gamma_fin>"
  Re1/1 -> Divide/1
  alpha_fin/1 -> Divide/2
  delta_fin/1 -> Divide/3
  gamma_fin/1 -> Divide/4
  Divide/1 -> Gain/1
  Re2/1 -> Divide1/1
  alpha_fin1/1 -> Divide1/2
  delta_fin1/1 -> Divide1/3
  gamma_fin1/1 -> Divide1/4
  Divide1/1 -> Gain1/1
  Constant8/1 -> Add/2
  Gain1/1 -> Add/1
  Add/1 -> gamma_fin2/1
  Constant9/1 -> gamma_fin2/2
  gamma_fin2/1 -> Divide2/2
  Gain/1 -> Divide2/1
  Divide2/1 -> Colburn_J_factor/1

== system PowerFlowLib/Energy & Power Systems/Thermal/ECS/Air-Air HX/Friction_factor_cold ==
  Fin_prameter_ratios : Inport
  Re : Inport  Port=2
  Add : Sum
  Bus Selector : BusSelector  OutputSignals=alpha_fin,delta_fin,gamma_fin
  Constant : Constant  Value=-0.7422
  Constant1 : Constant  Value=-0.1856
  Constant2 : Constant  Value=0.3053
  Constant3 : Constant  Value=-0.2659
  Constant4 : Constant  Value=4.429
  Constant5 : Constant  Value=0.92
  Constant6 : Constant  Value=3.767
  Constant7 : Constant  Value=0.236
  Constant8 : Constant
  Constant9 : Constant  Value=0.1
  Divide : Product  Inputs=****
  Divide1 : Product  Inputs=****
  Divide2 : Product  Inputs=**
  Gain : Gain  Gain=9.6243
  Gain1 : Gain  Gain=7.669*10^(-8)
  Re1 : Math  Operator=pow  SaturateOnIntegerOverflow=on
  Re2 : Math  Operator=pow  SaturateOnIntegerOverflow=on
  alpha_fin : Math  Operator=pow  SaturateOnIntegerOverflow=on
  alpha_fin1 : Math  Operator=pow  SaturateOnIntegerOverflow=on
  delta_fin : Math  Operator=pow  SaturateOnIntegerOverflow=on
  delta_fin1 : Math  Operator=pow  SaturateOnIntegerOverflow=on
  gamma_fin : Math  Operator=pow  SaturateOnIntegerOverflow=on
  gamma_fin1 : Math  Operator=pow  SaturateOnIntegerOverflow=on
  gamma_fin2 : Math  Operator=pow  SaturateOnIntegerOverflow=on
  Friction_factor : Outport
  wires:
  Fin_prameter_ratios/1 -> Bus Selector/1
  Constant/1 -> Re1/2
  Constant1/1 -> alpha_fin/2
  Constant2/1 -> delta_fin/2
  Constant3/1 -> gamma_fin/2
  Constant4/1 -> Re2/2
  Constant5/1 -> alpha_fin1/2
  Constant6/1 -> delta_fin1/2
  Constant7/1 -> gamma_fin1/2
  Re/1 -> Re1/1, Re2/1
  Bus Selector/1 -> alpha_fin/1, alpha_fin1/1  "<alpha_fin>"
  Bus Selector/2 -> delta_fin/1, delta_fin1/1  "<delta_fin>"
  Bus Selector/3 -> gamma_fin/1, gamma_fin1/1  "<gamma_fin>"
  Re1/1 -> Divide/1
  alpha_fin/1 -> Divide/2
  delta_fin/1 -> Divide/3
  gamma_fin/1 -> Divide/4
  Divide/1 -> Gain/1
  Re2/1 -> Divide1/1
  alpha_fin1/1 -> Divide1/2
  delta_fin1/1 -> Divide1/3
  gamma_fin1/1 -> Divide1/4
  Divide1/1 -> Gain1/1
  Constant8/1 -> Add/2
  Gain1/1 -> Add/1
  Add/1 -> gamma_fin2/1
  Constant9/1 -> gamma_fin2/2
  gamma_fin2/1 -> Divide2/2
  Gain/1 -> Divide2/1
  Divide2/1 -> Friction_factor/1

== system PowerFlowLib/Energy & Power Systems/Thermal/ECS/Air-Air HX/Friction_factor_hot ==
  Fin_prameter_ratios : Inport
  Re : Inport  Port=2
  Add : Sum
  Bus Selector : BusSelector  OutputSignals=alpha_fin,delta_fin,gamma_fin
  Constant : Constant  Value=-0.7422
  Constant1 : Constant  Value=-0.1856
  Constant2 : Constant  Value=0.3053
  Constant3 : Constant  Value=-0.2659
  Constant4 : Constant  Value=4.429
  Constant5 : Constant  Value=0.92
  Constant6 : Constant  Value=3.767
  Constant7 : Constant  Value=0.236
  Constant8 : Constant
  Constant9 : Constant  Value=0.1
  Divide : Product  Inputs=****
  Divide1 : Product  Inputs=****
  Divide2 : Product  Inputs=**
  Gain : Gain  Gain=9.6243
  Gain1 : Gain  Gain=7.669*10^(-8)
  Re1 : Math  Operator=pow  SaturateOnIntegerOverflow=on
  Re2 : Math  Operator=pow  SaturateOnIntegerOverflow=on
  alpha_fin : Math  Operator=pow  SaturateOnIntegerOverflow=on
  alpha_fin1 : Math  Operator=pow  SaturateOnIntegerOverflow=on
  delta_fin : Math  Operator=pow  SaturateOnIntegerOverflow=on
  delta_fin1 : Math  Operator=pow  SaturateOnIntegerOverflow=on
  gamma_fin : Math  Operator=pow  SaturateOnIntegerOverflow=on
  gamma_fin1 : Math  Operator=pow  SaturateOnIntegerOverflow=on
  gamma_fin2 : Math  Operator=pow  SaturateOnIntegerOverflow=on
  Friction_factor : Outport
  wires:
  Divide2/1 -> Friction_factor/1
  Gain/1 -> Divide2/1
  gamma_fin2/1 -> Divide2/2
  Constant9/1 -> gamma_fin2/2
  Add/1 -> gamma_fin2/1
  Gain1/1 -> Add/1
  Constant8/1 -> Add/2
  Divide1/1 -> Gain1/1
  gamma_fin1/1 -> Divide1/4
  delta_fin1/1 -> Divide1/3
  alpha_fin1/1 -> Divide1/2
  Re2/1 -> Divide1/1
  Divide/1 -> Gain/1
  gamma_fin/1 -> Divide/4
  delta_fin/1 -> Divide/3
  alpha_fin/1 -> Divide/2
  Re1/1 -> Divide/1
  Bus Selector/3 -> gamma_fin1/1, gamma_fin/1  "<gamma_fin>"
  Bus Selector/2 -> delta_fin1/1, delta_fin/1  "<delta_fin>"
  Bus Selector/1 -> alpha_fin1/1, alpha_fin/1  "<alpha_fin>"
  Re/1 -> Re2/1, Re1/1
  Constant7/1 -> gamma_fin1/2
  Constant6/1 -> delta_fin1/2
  Constant5/1 -> alpha_fin1/2
  Constant4/1 -> Re2/2
  Constant3/1 -> gamma_fin/2
  Constant2/1 -> delta_fin/2
  Constant1/1 -> alpha_fin/2
  Constant/1 -> Re1/2
  Fin_prameter_ratios/1 -> Bus Selector/1

== system PowerFlowLib/Energy & Power Systems/Thermal/ECS/Air-Air HX/HX_and_Fin_paramters ==
  Bus Creator1 : BusCreator  Inputs=6
  Bus Creator2 : BusCreator  Inputs=6
  Bus Creator3 : BusCreator  Inputs=3
  Fin_parameters : Subsystem
  HX_parameters : Subsystem
  Other_HX_parameters2 : Subsystem
  alpha : Product  Inputs=*/
  delta : Product  Inputs=*/
  gamma : Product  Inputs=*/
  HX_parameters2 : Outport
  Fin_parameters1 : Outport  Port=2
  Fin_parameters_ratios : Outport  Port=3
  wires:
  [Other_HX_parameters] -> HX_parameters/1(Other_HX_parameters)
  Other_HX_parameters2/1(Out1) -> [Other_HX_parameters]
  Bus Creator3/1 -> Fin_parameters_ratios/1
  gamma/1 -> Bus Creator3/3  "gamma_fin"
  delta/1 -> Bus Creator3/2  "delta_fin"
  alpha/1 -> Bus Creator3/1  "alpha_fin"
  Bus Creator1/1 -> HX_parameters2/1
  Bus Creator2/1 -> HX_parameters/2(Fin_parameters), Fin_parameters1/1
  HX_parameters/1(tot_free_flow_area_m^2) -> Bus Creator1/1  "A"
  Fin_parameters/3(Fin_free_flow_width_m) -> Bus Creator2/3, alpha/1, gamma/2  "s_fin"
  Fin_parameters/6(Fin_eff) -> Bus Creator2/6  "eta_fin"
  Fin_parameters/5(K_fin_Wm-1K-1) -> Bus Creator2/5  "K_n"
  Fin_parameters/4(Fin_free_flow_height_m) -> Bus Creator2/4, alpha/2  "h_fin"
  Fin_parameters/2(Fin_thickness_m) -> gamma/1, Bus Creator2/2, delta/1  "t_fin"
  Fin_parameters/1(Fin_length_m) -> Bus Creator2/1, delta/2  "l_fin"
  HX_parameters/6(m_hx_kg) -> Bus Creator1/6  "m_cm"
  HX_parameters/5(cp_hx_Jkg-1K-1) -> Bus Creator1/5  "cp_hx"
  HX_parameters/4(K_hx_Wm-1K-1) -> Bus Creator1/4  "K_p"
  HX_parameters/3(tot_no_of_fins_per_HX_per_flow) -> Bus Creator1/3  "N_f"
  HX_parameters/2(tot_length_in_direc_of_flow_m) -> Bus Creator1/2  "L_hx"

== system PowerFlowLib/Energy & Power Systems/Thermal/ECS/Air-Air HX/Heat_load_cold_side ==
  In_flow_bus : Inport
  air_properties : Inport  Port=2
  temp_out_degreeC : Inport  Port=3
  Bus Selector : BusSelector  OutputSignals=temp_C,mdot_kgps
  Bus Selector1 : BusSelector  OutputSignals=cp_air
  Product : Product  Inputs=3  RndMeth=Zero
  temp_diff : Sum  Inputs=-+
  Heat_rate_Watt : Outport
  wires:
  In_flow_bus/1 -> Bus Selector/1
  air_properties/1 -> Bus Selector1/1
  Bus Selector/1 -> temp_diff/1  "<temp_C>"
  temp_out_degreeC/1 -> temp_diff/2
  Bus Selector/2 -> Product/1  "<mdot_kgps>"
  Bus Selector1/1 -> Product/2  "<cp_air>"
  temp_diff/1 -> Product/3
  Product/1 -> Heat_rate_Watt/1

== system PowerFlowLib/Energy & Power Systems/Thermal/ECS/Air-Air HX/Heat_load_hot_side ==
  In_flow_bus : Inport
  air_properties : Inport  Port=2
  temp_out_degreeC : Inport  Port=3
  Bus Selector : BusSelector  OutputSignals=temp_C,mdot_kgps
  Bus Selector1 : BusSelector  OutputSignals=cp_air
  Product : Product  Inputs=3  RndMeth=Zero
  temp_diff : Sum  Inputs=+-
  Heat_rate_Watt : Outport
  wires:
  Product/1 -> Heat_rate_Watt/1
  temp_diff/1 -> Product/3
  Bus Selector1/1 -> Product/2  "<cp_air>"
  Bus Selector/2 -> Product/1  "<mdot_kgps>"
  temp_out_degreeC/1 -> temp_diff/2
  Bus Selector/1 -> temp_diff/1  "<temp_C>"
  air_properties/1 -> Bus Selector1/1
  In_flow_bus/1 -> Bus Selector/1

== system PowerFlowLib/Energy & Power Systems/Thermal/ECS/Air-Air HX/Hydraulic_diam_m ==
  Fin_parameters : Inport
  Add : Sum  Inputs=+++
  Add1 : Sum
  Bus Selector1 : BusSelector  OutputSignals=l_fin,t_fin,s_fin,h_fin,K_n,eta_fin
  Gain : Gain  Gain=4
  Gain1 : Gain  Gain=2
  Terminator : Terminator
  Terminator1 : Terminator
  hl : Product  Inputs=**
  shl : Product  Inputs=***
  sl : Product  Inputs=**
  th : Product  Inputs=**
  ts : Product  Inputs=**
  ts1 : Product  Inputs=*/
  Out1 : Outport
  wires:
  ts1/1 -> Out1/1
  Add1/1 -> ts1/2
  Gain/1 -> ts1/1
  ts/1 -> Add1/2
  Gain1/1 -> Add1/1
  Add/1 -> Gain1/1
  th/1 -> Add/3
  hl/1 -> Add/2
  sl/1 -> Add/1
  Bus Selector1/2 -> th/1, ts/1  "<t_fin>"
  shl/1 -> Gain/1
  Bus Selector1/1 -> hl/2, sl/2, shl/3  "<l_fin>"
  Bus Selector1/4 -> th/2, shl/2, hl/1  "<h_fin>"
  Bus Selector1/3 -> ts/2, sl/1, shl/1  "<s_fin>"
  Fin_parameters/1 -> Bus Selector1/1
  Bus Selector1/5 -> Terminator/1  "<K_n>"
  Bus Selector1/6 -> Terminator1/1  "<eta_fin>"

== system PowerFlowLib/Energy & Power Systems/Thermal/ECS/Air-Air HX/Pressure_drop_cold ==
  Friction_factor : Inport
  HX_parameters : Inport  Port=2
  air_properties : Inport  Port=3
  air_velocity : Inport  Port=4
  D_hydraulic : Inport  Port=5
  In_flow_bus : Inport  Port=6
  Add : Sum  Inputs=-+
  Bus Selector : BusSelector  OutputSignals=L_hx
  Bus Selector1 : BusSelector  OutputSignals=rho_air
  Bus Selector2 : BusSelector  OutputSignals=press_Pa
  Constant : Constant  Value=2
  Divide3 : Product  Inputs=****/
  Gain2 : Gain  Gain=2
  Math Function : Math  Operator=pow  SaturateOnIntegerOverflow=on
  pres_drop_Pa : Outport
  pres_Pa : Outport  Port=2
  wires:
  Friction_factor/1 -> Divide3/1
  HX_parameters/1 -> Bus Selector/1
  Bus Selector/1 -> Divide3/2  "<L_hx>"
  air_properties/1 -> Bus Selector1/1
  Bus Selector1/1 -> Divide3/3  "<rho_air>"
  air_velocity/1 -> Math Function/1
  Constant/1 -> Math Function/2
  Math Function/1 -> Divide3/4
  D_hydraulic/1 -> Divide3/5
  Divide3/1 -> Gain2/1
  Gain2/1 -> pres_drop_Pa/1, Add/1  "pres_drop_Pa"
  In_flow_bus/1 -> Bus Selector2/1
  Bus Selector2/1 -> Add/2  "<press_Pa>"
  Add/1 -> pres_Pa/1

== system PowerFlowLib/Energy & Power Systems/Thermal/ECS/Air-Air HX/Pressure_drop_hot ==
  Friction_factor : Inport
  HX_parameters : Inport  Port=2
  air_properties : Inport  Port=3
  air_velocity : Inport  Port=4
  D_hydraulic : Inport  Port=5
  In_flow_bus : Inport  Port=6
  Add : Sum  Inputs=-+
  Bus Selector : BusSelector  OutputSignals=L_hx
  Bus Selector1 : BusSelector  OutputSignals=rho_air
  Bus Selector2 : BusSelector  OutputSignals=pres_Pa
  Constant : Constant  Value=2
  Divide3 : Product  Inputs=****/
  Gain2 : Gain  Gain=2
  Math Function : Math  Operator=pow  SaturateOnIntegerOverflow=on
  pres_drop_Pa : Outport
  pres_Pa : Outport  Port=2
  wires:
  Add/1 -> pres_Pa/1
  Bus Selector2/1 -> Add/2  "<pres_Pa>"
  In_flow_bus/1 -> Bus Selector2/1
  Gain2/1 -> Add/1, pres_drop_Pa/1  "pres_drop_Pa"
  Divide3/1 -> Gain2/1
  D_hydraulic/1 -> Divide3/5
  Math Function/1 -> Divide3/4
  Constant/1 -> Math Function/2
  air_velocity/1 -> Math Function/1
  Bus Selector1/1 -> Divide3/3  "<rho_air>"
  air_properties/1 -> Bus Selector1/1
  Bus Selector/1 -> Divide3/2  "<L_hx>"
  HX_parameters/1 -> Bus Selector/1
  Friction_factor/1 -> Divide3/1

== system PowerFlowLib/Energy & Power Systems/Thermal/ECS/Air-Air HX/Re_number_in_cold ==
  In_flow_bus : Inport
  air_properties : Inport  Port=2
  Hydraulic_diam : Inport  Port=3
  HX_paramters : Inport  Port=4
  Bus Selector : BusSelector  OutputSignals=mdot_kgps
  Bus Selector1 : BusSelector  OutputSignals=rho_air,mu_air
  Bus Selector2 : BusSelector  OutputSignals=A
  Re_number_claculation : Product  Inputs=***/
  Velocity_calculation : Product  Inputs=*//
  Re_number : Outport
  velo_air_ms-1 : Outport  Port=2
  wires:
  air_properties/1 -> Bus Selector1/1
  In_flow_bus/1 -> Bus Selector/1
  HX_paramters/1 -> Bus Selector2/1
  Bus Selector/1 -> Velocity_calculation/1  "<mdot_kgps>"
  Bus Selector1/1 -> Velocity_calculation/2, Re_number_claculation/1  "<rho_air>"
  Bus Selector2/1 -> Velocity_calculation/3  "<A>"
  Velocity_calculation/1 -> velo_air_ms-1/1, Re_number_claculation/2  "Velo_air_ms-1"
  Hydraulic_diam/1 -> Re_number_claculation/3
  Bus Selector1/2 -> Re_number_claculation/4  "<mu_air>"
  Re_number_claculation/1 -> Re_number/1  "Re_number"

== system PowerFlowLib/Energy & Power Systems/Thermal/ECS/Air-Air HX/Re_number_in_hot ==
  In_flow_bus : Inport
  air_properties : Inport  Port=2
  Hydraulic_diam : Inport  Port=3
  HX_paramters : Inport  Port=4
  Bus Selector : BusSelector  OutputSignals=mdot_kgps
  Bus Selector1 : BusSelector  OutputSignals=rho_air,mu_air
  Bus Selector2 : BusSelector  OutputSignals=A
  Re_number_claculation : Product  Inputs=***/
  Velocity_calculation : Product  Inputs=*//
  Re_number : Outport
  velo_air_ms-1 : Outport  Port=2
  wires:
  Re_number_claculation/1 -> Re_number/1  "Re_number"
  Bus Selector1/2 -> Re_number_claculation/4  "<mu_air>"
  Hydraulic_diam/1 -> Re_number_claculation/3
  Velocity_calculation/1 -> velo_air_ms-1/1, Re_number_claculation/2  "Velo_air_ms-1"
  Bus Selector2/1 -> Velocity_calculation/3  "<A>"
  Bus Selector1/1 -> Re_number_claculation/1, Velocity_calculation/2  "<rho_air>"
  Bus Selector/1 -> Velocity_calculation/1  "<mdot_kgps>"
  HX_paramters/1 -> Bus Selector2/1
  In_flow_bus/1 -> Bus Selector/1
  air_properties/1 -> Bus Selector1/1

== system PowerFlowLib/Energy & Power Systems/Thermal/ECS/Air-Air HX/Thermal_resistance_KpW_cold ==
  Convective_HTC : Inport
  HX_parameters : Inport  Port=2
  Fin_parameters : Inport  Port=3
  Add : Sum
  Bus Selector : BusSelector  OutputSignals=N_f
  Bus Selector1 : BusSelector  OutputSignals=s_fin,l_fin,eta_fin,h_fin
  Calc_R_tot : Product  Inputs=**
  Calc_R_tot1 : Product  Inputs=*/
  Constant : Constant  Value=2
  Gain : Gain  Gain=2
  R1_Convection_to_plate/fin_base : Product  Inputs=////
  R1_convection_fin_or_plate_base_KpW : Display
  R5_Conv-conduction_through  fin_projection : Product  Inputs=//////
  R5_convection_fin_projection_KpW : Display
  R_tot_K/W : Outport
  wires:
  HX_parameters/1 -> Bus Selector/1
  Fin_parameters/1 -> Bus Selector1/1
  Convective_HTC/1 -> R1_Convection_to_plate/fin_base/1, R5_Conv-conduction_through  fin_projection/3  "HTC_Wpm2K"
  Bus Selector/1 -> R1_Convection_to_plate/fin_base/2, R5_Conv-conduction_through  fin_projection/4  "<N_f>"
  Bus Selector1/1 -> R1_Convection_to_plate/fin_base/3  "<s_fin>"
  Bus Selector1/2 -> R1_Convection_to_plate/fin_base/4, R5_Conv-conduction_through  fin_projection/6  "<l_fin>"
  R1_Convection_to_plate/fin_base/1 -> R1_convection_fin_or_plate_base_KpW/1, Calc_R_tot/1, Add/1
  Constant/1 -> R5_Conv-conduction_through  fin_projection/1
  Bus Selector1/3 -> R5_Conv-conduction_through  fin_projection/2  "<eta_fin>"
  Bus Selector1/4 -> R5_Conv-conduction_through  fin_projection/5  "<h_fin>"
  R5_Conv-conduction_through  fin_projection/1 -> R5_convection_fin_projection_KpW/1, Calc_R_tot/2, Gain/1
  Gain/1 -> Add/2
  Calc_R_tot/1 -> Calc_R_tot1/1  "R1R5"
  Add/1 -> Calc_R_tot1/2  "R1+2R5"
  Calc_R_tot1/1 -> R_tot_K/W/1  "Rtot"

== system PowerFlowLib/Energy & Power Systems/Thermal/ECS/Air-Air HX/Thermal_resistance_KpW_hot ==
  Convective_HTC : Inport
  HX_parameters : Inport  Port=2
  Fin_parameters : Inport  Port=3
  Add : Sum
  Bus Selector : BusSelector  OutputSignals=N_f
  Bus Selector1 : BusSelector  OutputSignals=s_fin,l_fin,eta_fin,h_fin
  Calc_R_tot : Product  Inputs=**
  Calc_R_tot1 : Product  Inputs=*/
  Constant : Constant  Value=2
  Gain : Gain  Gain=2
  R1_Convection_to_plate/fin_base : Product  Inputs=////
  R1_convection_fin_or_plate_base_KpW : Display
  R5_Conv-conduction_through  fin_projection : Product  Inputs=//////
  R5_convection_fin_projection_KpW : Display
  R_tot_K/W : Outport
  wires:
  Calc_R_tot1/1 -> R_tot_K/W/1  "Rtot"
  Add/1 -> Calc_R_tot1/2  "R1+2R5"
  Calc_R_tot/1 -> Calc_R_tot1/1  "R1R5"
  Gain/1 -> Add/2
  R5_Conv-conduction_through  fin_projection/1 -> Gain/1, Calc_R_tot/2, R5_convection_fin_projection_KpW/1
  Bus Selector1/4 -> R5_Conv-conduction_through  fin_projection/5  "<h_fin>"
  Bus Selector1/3 -> R5_Conv-conduction_through  fin_projection/2  "<eta_fin>"
  Constant/1 -> R5_Conv-conduction_through  fin_projection/1
  R1_Convection_to_plate/fin_base/1 -> Add/1, Calc_R_tot/1, R1_convection_fin_or_plate_base_KpW/1
  Bus Selector1/2 -> R5_Conv-conduction_through  fin_projection/6, R1_Convection_to_plate/fin_base/4  "<l_fin>"
  Bus Selector1/1 -> R1_Convection_to_plate/fin_base/3  "<s_fin>"
  Bus Selector/1 -> R5_Conv-conduction_through  fin_projection/4, R1_Convection_to_plate/fin_base/2  "<N_f>"
  Convective_HTC/1 -> R5_Conv-conduction_through  fin_projection/3, R1_Convection_to_plate/fin_base/1  "HTC_Wpm2K"
  Fin_parameters/1 -> Bus Selector1/1
  HX_parameters/1 -> Bus Selector/1

== system PowerFlowLib/Energy & Power Systems/Thermal/ECS/Air-Air HX/convective_HTC_Wm-2K-1_cold ==
  Colburn_J_factor : Inport
  Re : Inport  Port=2
  air_properties : Inport  Port=3
  hydraulic_diameter : Inport  Port=4
  Bus Selector : BusSelector  OutputSignals=Pr,K_air
  Constant : Constant  Value=1/3
  Divide : Product  Inputs=****/
  Math Function : Math  Operator=pow  SaturateOnIntegerOverflow=on
  Convective_HTC_Wm-2K-1 : Outport
  wires:
  air_properties/1 -> Bus Selector/1
  Colburn_J_factor/1 -> Divide/1
  Re/1 -> Divide/2
  Bus Selector/1 -> Math Function/1  "<Pr>"
  Constant/1 -> Math Function/2
  Math Function/1 -> Divide/3
  Bus Selector/2 -> Divide/4  "<K_air>"
  hydraulic_diameter/1 -> Divide/5
  Divide/1 -> Convective_HTC_Wm-2K-1/1
